simulink model "EIG_24Aprile"  (R2025b)
settings: Solver=VariableStepAuto  StartTime=0.0  StopTime=50.0  RelTol=1e-3
undefined symbols (not defined in the file): A, B, K_eig, N, n, x0_eig, xref
settings Model: Creator=salvo  LastModifiedBy=salvo

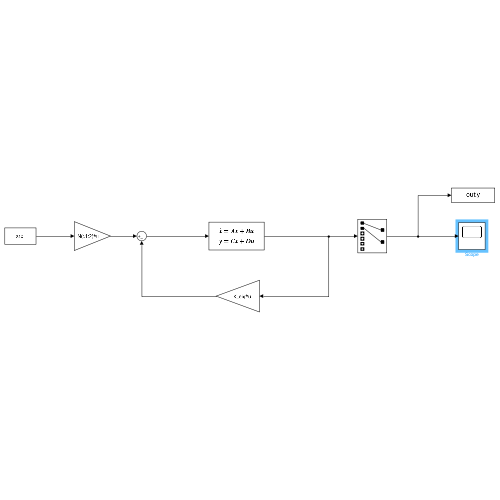
[thumbnail: Simulink's stored preview of the top-level diagram]
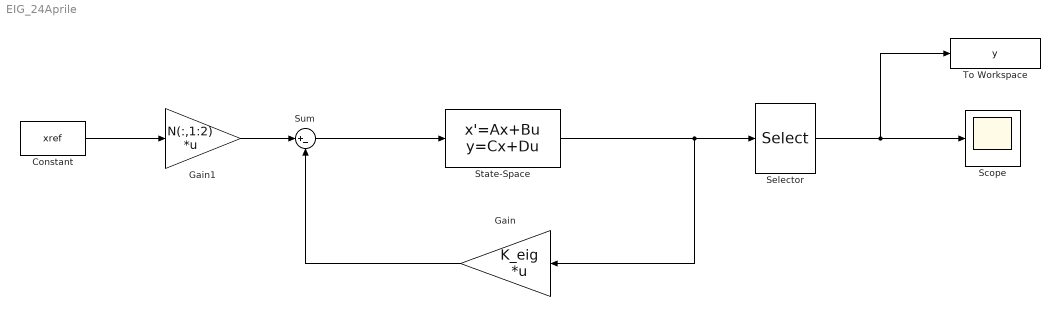
== system EIG_24Aprile ==
  Constant : Constant  Value=xref
  Gain : Gain  Gain=K_eig  Multiplication=Matrix(K*u)
  Gain1 : Gain  Gain=N(:,1:2)  Multiplication=Matrix(K*u)
  Scope : Scope
      settings: ActiveDisplayYMinimum=0.11087922310941128  ActiveDisplayYMaximum=0.18334912258630867
  Selector : Selector  InputPortWidth=6  IndexOptions=Index vector (dialog)  Indices=[1 2 ]  OutputSizes=1
  State-Space : StateSpace  A=A  B=B  C=eye(n)  D=zeros(6,2)  InitialCondition=[x0_eig; zeros(3,1)]
  Sum : Sum  Inputs=|+-
  To Workspace : ToWorkspace  VariableName=y  SaveFormat=Timeseries  SampleTime=-1
  wires:
  State-Space/1 -> Gain/1, Selector/1
  Selector/1 -> To Workspace/1, Scope/1
  Gain/1 -> Sum/2
  Sum/1 -> State-Space/1
  Constant/1 -> Gain1/1
  Gain1/1 -> Sum/1
